simulink model "Common_Rail_CRDI"  (R2019a)
settings: Solver=FixedStepDiscrete  StartTime=0.0  StopTime=10.0  FixedStep=0.01  RelTol=1e-3
settings Model: Creator=user  LastModifiedBy=user
settings ConfigComp: DVTestSuiteOptimization=Auto  DVDetectDeadLogic=on  DVDetectOutOfBounds=on  DVRebuildModelRepresentation=Always

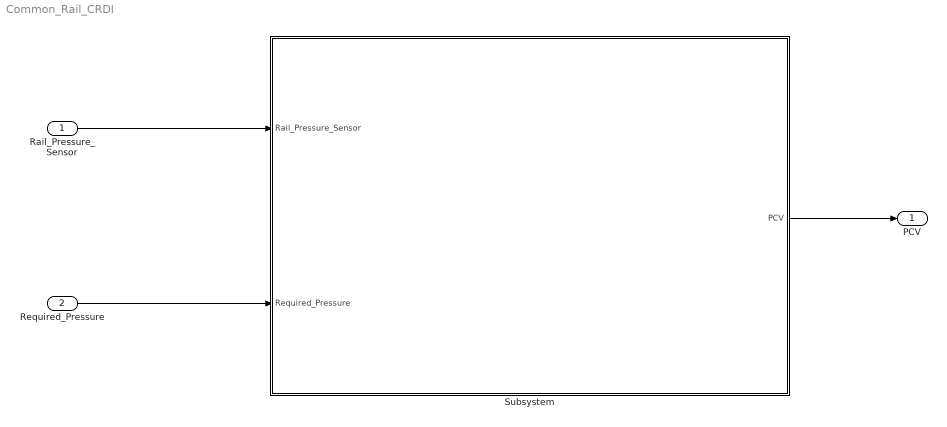
== system Common_Rail_CRDI ==
  Rail_Pressure_Sensor : Inport
  Required_Pressure : Inport  Port=2
  Subsystem : Subsystem  TreatAsAtomicUnit=on
  PCV : Outport
  wires:
  Rail_Pressure_Sensor/1 -> Subsystem/1(Rail_Pressure_Sensor)
  Required_Pressure/1 -> Subsystem/2(Required_Pressure)
  Subsystem/1(PCV) -> PCV/1

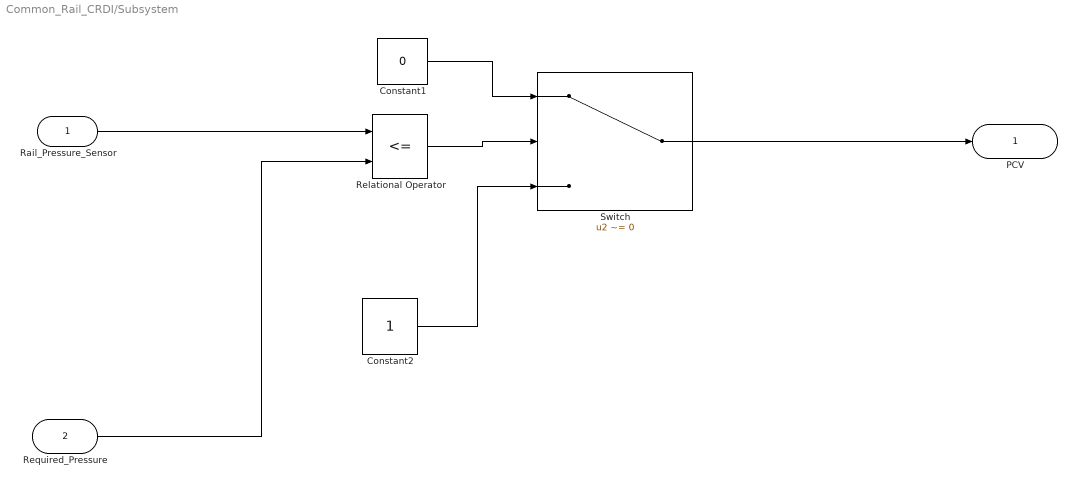
== system Common_Rail_CRDI/Subsystem ==
  Rail_Pressure_Sensor : Inport  OutDataTypeStr=uint16
  Required_Pressure : Inport  Port=2  OutDataTypeStr=uint16
  Constant1 : Constant  Value=0  OutDataTypeStr=int8
  Constant2 : Constant  OutDataTypeStr=int8
  Relational Operator : RelationalOperator  Operator=<=  OutDataTypeStr=boolean  RndMeth=Simplest
  Switch : Switch  Criteria=u2 ~= 0  OutDataTypeStr=boolean
  PCV : Outport  OutDataTypeStr=boolean
  wires:
  Required_Pressure/1 -> Relational Operator/2
  Relational Operator/1 -> Switch/2
  Rail_Pressure_Sensor/1 -> Relational Operator/1
  Constant1/1 -> Switch/1
  Switch/1 -> PCV/1
  Constant2/1 -> Switch/3
